simulink model "untitled"  (R2023a)
settings: Solver=VariableStepAuto  StartTime=0.0  StopTime=10.0  RelTol=1e-3
values from neighbouring files (symbols this model uses):
  b_eq = b_eq_max    [FrecuenciaNatural_Amortiguamiento.m]    (also in variables.m = 2.19444444444e-05)
  g = 9.80665    [variables.m]
  J_eq = J_eq_max    [FrecuenciaNatural_Amortiguamiento.m]    (also in variables.m = 4.58263888889e-05)
  k_l = m*l_cm + m_l*l_l    (= 1)    [variables.m]
  Pp = 3    [variables.m]
  r = 120    [esp_de_operacion.m]    (also in variables.m)
settings Model: Creator=Juan  LastModifiedBy=Juan

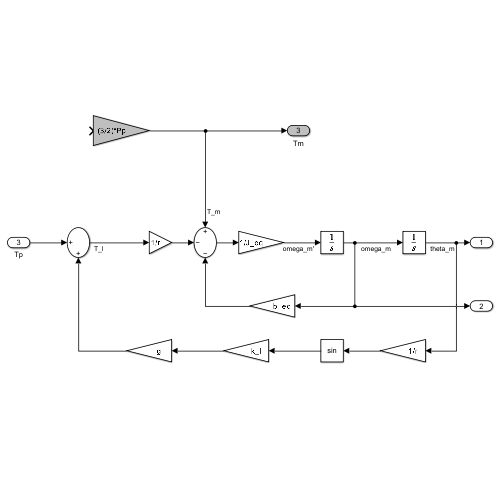
[thumbnail: Simulink's stored preview of the top-level diagram]
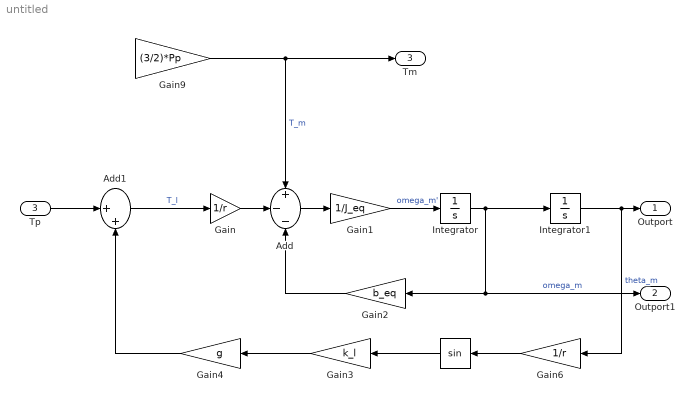
== system untitled ==
  Tp : Inport  Port=3
  " " : Trigonometry
  Add : Sum  Inputs=+--
  Add1 : Sum  Inputs=|++
  Gain : Gain  Gain=1/r
  Gain1 : Gain  Gain=1/J_eq
  Gain2 : Gain  Gain=b_eq
  Gain3 : Gain  Gain=k_l
  Gain4 : Gain  Gain=g
  Gain6 : Gain  Gain=1/r
  Gain9 : Gain  Gain=(3/2)*Pp
  Integrator : Integrator
  Integrator1 : Integrator
  Outport : Outport
  Outport1 : Outport  Port=2
  Tm : Outport  Port=3
  wires:
  Gain/1 -> Add/2
  Add/1 -> Gain1/1
  Gain2/1 -> Add/3
  Gain1/1 -> Integrator/1  "omega_m'"
  Integrator/1 -> Integrator1/1, Gain2/1, Outport1/1  "omega_m"
  Integrator1/1 -> Gain6/1, Outport/1  "theta_m"
  Gain3/1 -> Gain4/1
  " "/1 -> Gain3/1
  Gain4/1 -> Add1/2
  Tp/1 -> Add1/1
  Gain6/1 -> " "/1
  Add1/1 -> Gain/1  "T_l"
  Gain9/1 -> Tm/1, Add/1  "T_m"
